simulink model "diabetes_4mpc"  (R2019a)
settings: Solver=ode45  StartTime=0.0  StopTime=24  RelTol=1e-3  EnableMultiTasking=on
StopFcn:
  | plot_results
libraries: simulink x1
settings Model: Creator=tsladeche  LastModifiedBy=esthe
settings DataIOCC: LimitDataPoints=on  SaveFormat=Array  SignalLoggingSaveFormat=ModelDataLogs  ReturnWorkspaceOutputs=off
settings OptimizationCC: ExpressionDepthLimit=2147483647  LifeSpan=inf
settings DebuggingCC: UnderspecifiedInitializationDetection=Classic  MergeDetectMultiDrivingBlocksExec=none  SolverPrmCheckMsg=warning  FcnCallInpInsideContextMsg=warning  StateNameClashWarn=warning  SFUnexpectedBacktrackingDiag=warning  SFNoUnconditionalDefaultTransitionDiag=warning  SFExecutionAtInitializationDiag=none  ArithmeticOperatorsInVariantConditions=warning
settings HardwareCC: ProdBitPerPointer=32  ProdBitPerSizeT=32  ProdBitPerPtrDiffT=32  ProdLargestAtomicFloat=None  ProdIntDivRoundTo=Undefined  ProdEndianess=Unspecified  ProdWordSize=32  ProdHWDeviceType=32-bit Generic
settings ModelReferenceCC: PropagateSignalLabelsOutOfModel=off
settings SFSimCC: SimUseLocalCustomCode=off
settings RTWCC: RTWUseLocalCustomCode=off
settings CodeAppCC: StateflowObjectComments=on
settings GRTTargetCC: TargetLangStandard=C89/C90 (ANSI)  GeneratePreprocessorConditionals=Disable all  CombineOutputUpdateFcns=off  GRTInterface=on
settings ConfigComp: CovMetricSettings=dw  CovHtmlReporting=on  CovSaveCumulativeToWorkspaceVar=on  CovSaveSingleToWorkspaceVar=on  CovExternalEMLEnable=off

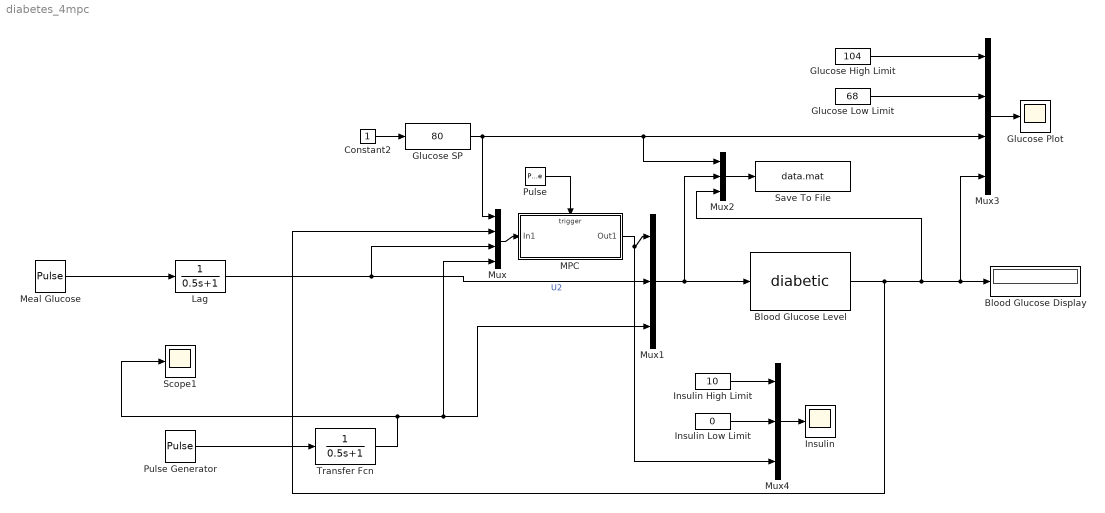
== system diabetes_4mpc ==
  Blood Glucose Display : Display
  Blood Glucose Level : S-Function  FunctionName=diabetic  SFunctionDeploymentMode=off  EnableBusSupport=off
  Constant2 : Constant
  Glucose High Limit : Constant  Value=104
  Glucose Low Limit : Constant  Value=68
  Glucose Plot : Scope
  Glucose SP : simulink/Math Operations/Slider Gain  gain=80  low=50  high=120
  Insulin : Scope
  Insulin High Limit : Constant  Value=10
  Insulin Low Limit : Constant  Value=0
  Lag : TransferFcn  Denominator=[0.5 1]
  MPC : Subsystem  TreatAsAtomicUnit=on
  Meal Glucose : DiscretePulseGenerator  PulseType=Time based  Amplitude=100  Period=6  PulseWidth=10  PhaseDelay=7
  Mux : Mux
  Mux1 : Mux  Inputs=3
  Mux2 : Mux  Inputs=3
  Mux3 : Mux
  Mux4 : Mux  Inputs=3
  Pulse : DiscretePulseGenerator  PulseType=Time based  Period=0.2  PulseWidth=5
  Pulse Generator : DiscretePulseGenerator  PulseType=Time based  Amplitude=50  Period=24  PulseWidth=6  PhaseDelay=5
  Save To File : ToFile  Filename=data.mat  MatrixName=diabetic  SampleTime=0.05
  Scope1 : Scope
  Transfer Fcn : TransferFcn  Denominator=[0.5 1]
  wires:
  Mux2/1 -> Save To File/1
  Mux1/1 -> Mux2/2, Blood Glucose Level/1
  Constant2/1 -> Glucose SP/1
  Glucose SP/1 -> Mux/1, Mux3/3, Mux2/1
  Blood Glucose Level/1 -> Mux/2, Mux3/4, Blood Glucose Display/1, Mux2/3
  Glucose High Limit/1 -> Mux3/1
  Glucose Low Limit/1 -> Mux3/2
  Mux3/1 -> Glucose Plot/1
  MPC/1(Out1) -> Mux4/3, Mux1/1
  Insulin High Limit/1 -> Mux4/1
  Insulin Low Limit/1 -> Mux4/2
  Mux4/1 -> Insulin/1
  Mux/1 -> MPC/1(In1)
  Pulse/1 -> MPC/Trigger
  Transfer Fcn/1 -> Mux/4, Mux1/3, Scope1/1
  Pulse Generator/1 -> Transfer Fcn/1
  Meal Glucose/1 -> Lag/1
  Lag/1 -> Mux/3, Mux1/2  "U2"

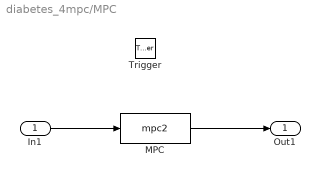
== system diabetes_4mpc/MPC ==
  In1 : Inport
  Trigger : TriggerPort  VariantControl=(inherit)
  MPC : MATLABFcn  MATLABFcn=mpc2
  Out1 : Outport
  wires:
  In1/1 -> MPC/1
  MPC/1 -> Out1/1
